simulink model "MSREPrimaryLoop_PlantLevel"  (R2024a)
settings: Solver=VariableStepAuto  StartTime=0.0  StopTime=500000  MaxStep=0.1  RelTol=1e-3
undefined symbols (not defined in the file): a_f, a_g, axialFuelImportance, axialGraphiteImportance, axialPowerFraction, beta, beta_t, bubbleSaturationLevel, bypassRatio, C0, coolantPHXChannelLength, coolantPHXDh, coolantPHXFlowArea, coreCorrectionNominalFlowRate, coreDowncomerArea, coreDowncomerHydraulicDiameter, coreDowncomerLength, coreDowncomerVolume, coreFlowArea, coreFuelVolume, coreInletFlowDistributerArea, coreInletFlowDistributerHydralicDiameter, coreInletFlowDistributerLength, coreInletFlowDistributerVolume, coreLowerPlenumArea, coreLowerPlenumHydraulicDiameter, coreLowerPlenumLength, coreLowerPlenumVolume, coreUpperPlenumArea, coreUpperPlenumLength, coreUpperPlenumVolume, coreVolume, cpGraphite, day, decayScale, decaySSFraction, dissolusionRatio, dMin, dScale, dsmConst, DXeG, externalReactivity, Fiss_factor, fuelChannelHydrualicDiameter, fuelChannelLength, fuelDepositRatio, fuelFraction, fuelGraphiteArea, fuelGraphiteHeatTransferCoefficient, gamma0, gamma1, gamma2, gasExchangeRatio, gasMixingEfficiency, gasPurgeRate, gasStrippingEfficiency, graphiteKDiff, graphiteUnitCellThickness, initialIodineConcentration, InitialXeMolarConcentration ... (+66)
libraries: fl_lib x291, nesl_utility x101, SimscapeFluids_lib x24, simulink x5, slpidlib x1
(part 5 of 13)

== system MSREPrimaryLoop_PlantLevel/Pump MSRE/Pump/PumpPysical ==
  XeIn : Inport
  GasIn : Inport  Port=2
  Add : Sum  Inputs=|++
  Delay One Step : Delay  DelayLength=1
  Gain : Gain  Gain=0.5
  GasCalc : Subsystem
      settings: PortSchema="{\"entries\":[{\"content\":{\"sides\":[{\"content\":{\"connectorIds\":[\"In1\"]},\"type\":\"ConnectorPlacement.EquallySpacedRectSide\",\"uuid\":\"a8e1ce06-71c9-462d-8d5c-7a3e078b5544\"},{\"content\":{\"connectorIds\":[\"Out1\"],\"side\":\"RIGHT\"},\"type\":\"ConnectorPlacement.EquallySpacedRectSide\",\"uuid\":\"2c63a1ce-15e2-4b17-a432-f9f40781bd58\"},{\"content\":{\"connectorIds\":[\"LConn1\",\"LConn2\",\"LConn3\"],\"side\":\"TOP\"},\"type\":\"ConnectorPlacement.EquallySpacedRectSide\",\"uuid\":\"abc20e07-15eb-475f-be7f-cc96378523a1\"},{\"content\":{\"connectorIds\":[],\"side\":\"BOTTOM\"},\"type\":\"ConnectorPlacement.EquallySpacedRectSide\",\"uuid\":\"ab58f362-f4c2-4e86-bda0-802426066295\"}]},\"type\":\"ConnectorPlacement.EquallySpacedConnector\",\"uuid\":\"b54d49a9-048b-4912-bf18-92a7ef5e8aff\"}],\"packageUris\":[\"http://schema.mathworks.com/mf0/Connector/R2020b\"],\"version\":\"1.0\"}"
  PumpPhysics&Control : Subsystem
      settings: PortSchema="{\"entries\":[{\"content\":{\"sides\":[{\"content\":{\"connectorIds\":[\"LConn1\",\"In1\"]},\"type\":\"ConnectorPlacement.EquallySpacedRectSide\",\"uuid\":\"dfa2aa95-b0f6-4d42-b52c-ac64f68b4332\"},{\"content\":{\"connectorIds\":[\"RConn1\"],\"side\":\"RIGHT\"},\"type\":\"ConnectorPlacement.EquallySpacedRectSide\",\"uuid\":\"4e233f45-275b-4a62-b54f-a26261252d76\"},{\"content\":{\"connectorIds\":[],\"side\":\"TOP\"},\"type\":\"ConnectorPlacement.EquallySpacedRectSide\",\"uuid\":\"4d56cee6-54c9-4b53-b595-9dd9843d1812\"},{\"content\":{\"connectorIds\":[\"RConn2\"],\"side\":\"BOTTOM\"},\"type\":\"ConnectorPlacement.EquallySpacedRectSide\",\"uuid\":\"5b59abd0-5c01-4c9b-8b33-a5a665899d43\"}]},\"type\":\"ConnectorPlacement.EquallySpacedConnector\",\"uuid\":\"08118153-6206-4ac8-9187-5e3d4b128de1\"}],\"packageUris\":[\"http://schema.mathworks.com/mf0/Connector/R2020b\"],\"version\":\"1.0\"}"
  XenonCalc : Subsystem
      settings: PortSchema="{\"entries\":[{\"content\":{\"sides\":[{\"content\":{\"connectorIds\":[\"In1\"]},\"type\":\"ConnectorPlacement.EquallySpacedRectSide\",\"uuid\":\"2d0a178d-e3ce-4b60-98e7-1a8cc2d8e60a\"},{\"content\":{\"connectorIds\":[\"Out1\"],\"side\":\"RIGHT\"},\"type\":\"ConnectorPlacement.EquallySpacedRectSide\",\"uuid\":\"c836f1a2-1f60-4759-a54a-d13020949774\"},{\"content\":{\"connectorIds\":[\"LConn1\"],\"side\":\"TOP\"},\"type\":\"ConnectorPlacement.EquallySpacedRectSide\",\"uuid\":\"88d5b9ac-da0a-4ad3-844b-69cd646a8f29\"},{\"content\":{\"connectorIds\":[],\"side\":\"BOTTOM\"},\"type\":\"ConnectorPlacement.EquallySpacedRectSide\",\"uuid\":\"7af8c1ea-1928-402f-ba73-00fd41d484c9\"}]},\"type\":\"ConnectorPlacement.EquallySpacedConnector\",\"uuid\":\"10dc3dbd-7ee0-472f-a356-245132d02761\"}],\"packageUris\":[\"http://schema.mathworks.com/mf0/Connector/R2020b\"],\"version\":\"1.0\"}"
  Inlet : PMIOPort  Side=Left
  Outlet : PMIOPort  Port=2  Side=Right
  XeOut : Outport
  GasOut : Outport  Port=2
  wires:
  GasIn/1 -> GasCalc/1(GasIn), Add/1
  GasCalc/1(GasOut) -> GasOut/1, Add/2
  Add/1 -> Gain/1
  Gain/1 -> Delay One Step/1
  Delay One Step/1 -> PumpPhysics&Control/1(GasRef)
  XeIn/1 -> XenonCalc/1(XeIn)
  XenonCalc/1(XeOut) -> XeOut/1
  connections:
  Inlet/RConn1 -- GasCalc/LConn1 -- PumpPhysics&Control/LConn1
  Outlet/RConn1 -- PumpPhysics&Control/RConn1 -- GasCalc/LConn3
  PumpPhysics&Control/RConn2 -- GasCalc/LConn2 -- XenonCalc/LConn1

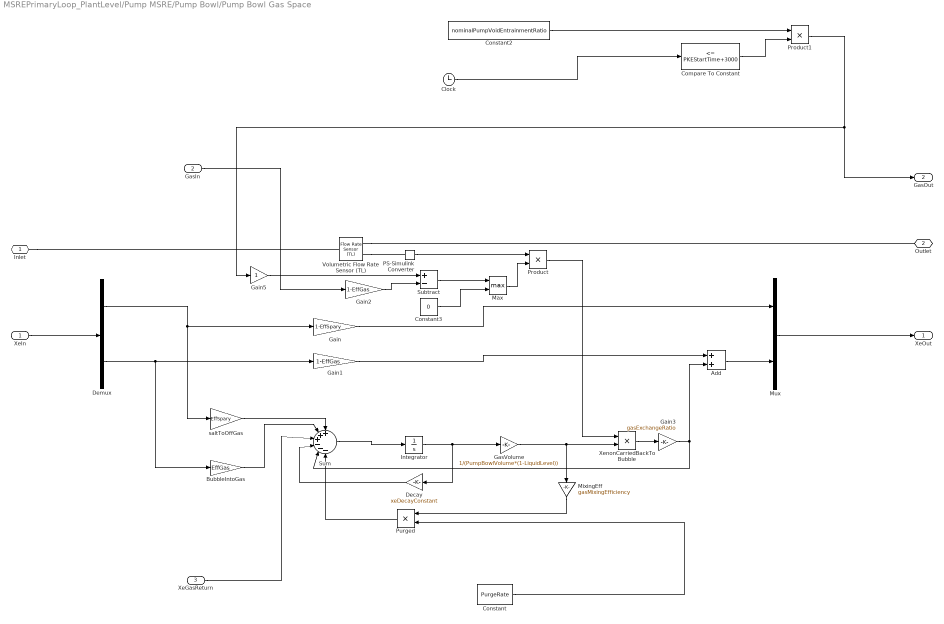
== system MSREPrimaryLoop_PlantLevel/Pump MSRE/Pump Bowl/Pump Bowl Gas Space ==
  XeIn : Inport  OutDataTypeStr=double  Unit=kg/s
  GasIn : Inport  Port=2
  XeGasReturn : Inport  Port=3
  Add : Sum
  BubbleIntoGas : Gain  Gain=EffGas
  Clock : Clock
  Compare To Constant : simulink/Logic and Bit Operations/Compare To Constant  relop=<=  const=PKEStartTime+3000  OutDataTypeStr=boolean
  Constant : Constant  Value=PurgeRate
  Constant2 : Constant  Value=nominalPumpVoidEntrainmentRatio
  Constant3 : Constant  Value=0
  Decay : Gain  Gain=xeDecayConstant
  Demux : Demux  Outputs=2
  Gain : Gain  Gain=1-EffSpary
  Gain1 : Gain  Gain=1-EffGas
  Gain2 : Gain  Gain=1-EffGas
  Gain3 : Gain  Gain=gasExchangeRatio
  Gain5 : Gain
  GasVolume : Gain  Gain=1/(PumpBowlVolume*(1-LiquidLevel))
  Integrator : Integrator  LimitOutput=on  LowerSaturationLimit=0
  Max : MinMax  Function=max  Inputs=2
  MixingEff : Gain  Gain=gasMixingEfficiency
  Mux : Mux  Inputs=2
  PS-Simulink Converter : nesl_utility/PS-Simulink Converter  PhysicalDomain=network_engine_domain  SubClassName=ps_output  LeftPortType=input  RightPortType=output  PseudoPeriodic=off  Frequencies=[]  VectorFormat=1-D array  Unit=inherit  AffineConversion=off
  Product : Product
  Product1 : Product
  Purged : Product
  Subtract : Sum  Inputs=+-
  Sum : Sum  Inputs=+++---
  Volumetric Flow Rate Sensor (TL) : fl_lib/Thermal Liquid/Sensors/Flow Rate Sensor (TL)  mass_flow_measure=false  volumetric_flow_measure=true  energy_flow_measure=false
      settings: InternalSimscapePortConfiguration="{\"Bottom\":[],\"Left\":[{\"id\":\"A\",\"label\":\"A\",\"type\":\"foundation.thermal_liquid.thermal_liquid\"}],\"Right\":[{\"id\":\"B\",\"label\":\"B\",\"type\":\"foundation.thermal_liquid.thermal_liquid\"},{\"id\":\"V\",\"label\":\"V\",\"type\":\"output\"}],\"Top\":[]}"
  XenonCarriedBackToBubble : Product
  saltToOffGas : Gain  Gain=EffSpary
  Inlet : PMIOPort  Side=Left
  Outlet : PMIOPort  Port=2  Side=Right
  XeOut : Outport
  GasOut : Outport  Port=2
  wires:
  XeIn/1 -> Demux/1
  Demux/2 -> Gain1/1, BubbleIntoGas/1
  Mux/1 -> XeOut/1
  Demux/1 -> saltToOffGas/1, Gain/1
  saltToOffGas/1 -> Sum/1
  BubbleIntoGas/1 -> Sum/2
  Integrator/1 -> Decay/1, GasVolume/1
  GasVolume/1 -> XenonCarriedBackToBubble/2, MixingEff/1
  MixingEff/1 -> Purged/1
  Sum/1 -> Integrator/1
  Decay/1 -> Sum/4
  Gain/1 -> Mux/1
  PS-Simulink Converter/1 -> Product/1
  Product/1 -> XenonCarriedBackToBubble/1
  GasIn/1 -> Gain2/1
  Gain1/1 -> Add/1
  Add/1 -> Mux/2
  Product1/1 -> Gain5/1, GasOut/1
  Gain2/1 -> Subtract/2
  Purged/1 -> Sum/6
  XeGasReturn/1 -> Sum/3
  XenonCarriedBackToBubble/1 -> Gain3/1
  Gain3/1 -> Add/2, Sum/5
  Gain5/1 -> Subtract/1
  Subtract/1 -> Max/1
  Max/1 -> Product/2
  Constant3/1 -> Max/2
  Constant/1 -> Purged/2
  Compare To Constant/1 -> Product1/2
  Clock/1 -> Compare To Constant/1
  Constant2/1 -> Product1/1
  connections:
  Inlet/RConn1 -- Volumetric Flow Rate Sensor (TL)/LConn1
  Volumetric Flow Rate Sensor (TL)/RConn1 -- Outlet/RConn1
  Volumetric Flow Rate Sensor (TL)/RConn2 -- PS-Simulink Converter/LConn1

== system MSREPrimaryLoop_PlantLevel/Pump MSRE/Pump Bowl/Salt Space ==
  XeIn : Inport
  GasIn : Inport  Port=2
  Clock : Clock
  Compare To Constant : simulink/Logic and Bit Operations/Compare To Constant  relop=<=  const=PKEStartTime+3000  OutDataTypeStr=boolean
  Constant : Constant  Value=nominalPumpVoidDischargeRatio
  Constant Volume Chamber (TL) : fl_lib/Thermal Liquid/Elements/Constant Volume Chamber (TL)  volume=PumpBowlVolume*LiquidLevel m^3  num_ports=foundation.enum.num_ports.two  area_A=1 m^2  area_B=1 m^2  area_C=0.01 m^2  area_D=0.01 m^2  p_I_specify=on  p_I_priority=High  p_I=P0 Pa  p_I_nominal_specify=off  p_I_nominal_value=1  p_I_nominal_unit=MPa  T_I_specify=on  T_I_priority=None  T_I=T0 K  T_I_nominal_specify=off  T_I_nominal_value=1  T_I_nominal_unit=K  u_I_specify=on  u_I_priority=None  u_I=cpMSRE J/kg  u_I_nominal_specify=off  u_I_nominal_value=1  u_I_nominal_unit=kJ/kg  rho_I_specify=on  rho_I_priority=None  rho_I=nominalFuelDensity kg/m^3  rho_I_nominal_specify=off  rho_I_nominal_value=1  rho_I_nominal_unit=kg/m^3
      settings: InternalSimscapePortConfiguration="{\"Bottom\":[],\"Left\":[{\"id\":\"A\",\"label\":\"A\",\"type\":\"foundation.thermal_liquid.thermal_liquid\"},{\"id\":\"H\",\"label\":\"H\",\"type\":\"foundation.thermal.thermal\"}],\"Right\":[{\"id\":\"B\",\"label\":\"B\",\"type\":\"foundation.thermal_liquid.thermal_liquid\"}],\"Top\":[]}"
  GasCalc : Subsystem  mask{PipeVolume=PumpBowlVolume*LiquidLevel}
      mask prompts: PipeVolume "Volume"
      settings: PortSchema="{\"entries\":[{\"content\":{\"sides\":[{\"content\":{\"connectorIds\":[\"In1\"]},\"type\":\"ConnectorPlacement.EquallySpacedRectSide\",\"uuid\":\"a8e1ce06-71c9-462d-8d5c-7a3e078b5544\"},{\"content\":{\"connectorIds\":[\"Out1\"],\"side\":\"RIGHT\"},\"type\":\"ConnectorPlacement.EquallySpacedRectSide\",\"uuid\":\"2c63a1ce-15e2-4b17-a432-f9f40781bd58\"},{\"content\":{\"connectorIds\":[\"LConn1\"],\"side\":\"TOP\"},\"type\":\"ConnectorPlacement.EquallySpacedRectSide\",\"uuid\":\"abc20e07-15eb-475f-be7f-cc96378523a1\"},{\"content\":{\"connectorIds\":[],\"side\":\"BOTTOM\"},\"type\":\"ConnectorPlacement.EquallySpacedRectSide\",\"uuid\":\"ab58f362-f4c2-4e86-bda0-802426066295\"}]},\"type\":\"ConnectorPlacement.EquallySpacedConnector\",\"uuid\":\"b54d49a9-048b-4912-bf18-92a7ef5e8aff\"}],\"packageUris\":[\"http://schema.mathworks.com/mf0/Connector/R2020b\"],\"version\":\"1.0\"}"
  Perfect Insulator : fl_lib/Thermal/Thermal Elements/Perfect Insulator  T_specify=off  T_priority=None  T=0 K  T_nominal_specify=off  T_nominal_value=1  T_nominal_unit=K
  Product1 : Product
  Volumetric Flow Rate Sensor (TL) : fl_lib/Thermal Liquid/Sensors/Flow Rate Sensor (TL)  mass_flow_measure=false  volumetric_flow_measure=true  energy_flow_measure=false
      settings: InternalSimscapePortConfiguration="{\"Bottom\":[],\"Left\":[{\"id\":\"A\",\"label\":\"A\",\"type\":\"foundation.thermal_liquid.thermal_liquid\"}],\"Right\":[{\"id\":\"B\",\"label\":\"B\",\"type\":\"foundation.thermal_liquid.thermal_liquid\"},{\"id\":\"V\",\"label\":\"V\",\"type\":\"output\"}],\"Top\":[]}"
  XenonCalcBowl : Subsystem  mask{PipeVolume=PumpBowlVolume*LiquidLevel, dsm=0.005*dScale, km=0.0001}
      mask prompts: PipeVolume "Volume"; dsm "Sauter Mean Diameter"; km "Mass Transfer Coefficient"
      settings: PortSchema="{\"entries\":[{\"content\":{\"sides\":[{\"content\":{\"connectorIds\":[\"LConn1\",\"In1\",\"In2\"]},\"type\":\"ConnectorPlacement.EquallySpacedRectSide\",\"uuid\":\"82f8e7e7-fd89-4597-952e-64db268d0190\"},{\"content\":{\"connectorIds\":[\"RConn1\",\"Out1\",\"Out2\"],\"side\":\"RIGHT\"},\"type\":\"ConnectorPlacement.EquallySpacedRectSide\",\"uuid\":\"4b3edad1-18f8-43fa-96ee-a24bb3384b59\"},{\"content\":{\"connectorIds\":[],\"side\":\"TOP\"},\"type\":\"ConnectorPlacement.EquallySpacedRectSide\",\"uuid\":\"43d4f51d-f841-40d6-804e-7f238a90dabe\"},{\"content\":{\"connectorIds\":[],\"side\":\"BOTTOM\"},\"type\":\"ConnectorPlacement.EquallySpacedRectSide\",\"uuid\":\"350f2274-4108-4e6e-a637-0ae7118de3f0\"}]},\"type\":\"ConnectorPlacement.EquallySpacedConnector\",\"uuid\":\"d7e795ea-9d5d-4a8c-83ab-dab42197cc2f\"}],\"packageUris\":[\"http://schema.mathworks.com/mf0/Connector/R2020b\"],\"version\":\"1.0\"}"
  Inlet : PMIOPort  Side=Left
  Outlet : PMIOPort  Port=2  Side=Right
  XeOut : Outport
  GasOut : Outport  Port=2
  XeGasReturn : Outport  Port=3
  wires:
  XeIn/1 -> XenonCalcBowl/1(XeIn)
  XenonCalcBowl/1(XeOut) -> XeOut/1
  GasIn/1 -> GasCalc/1(GasIn)
  GasCalc/1(AverageVoid) -> XenonCalcBowl/2(GasVoid)
  XenonCalcBowl/2(XeGasReturn) -> XeGasReturn/1
  Product1/1 -> GasOut/1
  Compare To Constant/1 -> Product1/2
  Clock/1 -> Compare To Constant/1
  Constant/1 -> Product1/1
  connections:
  XenonCalcBowl/LConn1 -- Volumetric Flow Rate Sensor (TL)/RConn1
  Volumetric Flow Rate Sensor (TL)/LConn1 -- Inlet/RConn1
  XenonCalcBowl/RConn1 -- Constant Volume Chamber (TL)/LConn1
  Constant Volume Chamber (TL)/RConn1 -- Outlet/RConn1
  Perfect Insulator/LConn1 -- Constant Volume Chamber (TL)/LConn2
  GasCalc/LConn1 -- Volumetric Flow Rate Sensor (TL)/RConn2

== system MSREPrimaryLoop_PlantLevel/Pump MSRE/Pump Flow Distribution/Subsystem1 ==
  note: Handle divide by zero.
  MainXeRate : fl_lib/Physical Signals/Functions/PS Divide
  Mass & Energy Flow Rate Sensor (TL) : fl_lib/Thermal Liquid/Sensors/Flow Rate Sensor (TL)  mass_flow_measure=true  volumetric_flow_measure=false  energy_flow_measure=true
      settings: InternalSimscapePortConfiguration="{\"Bottom\":[{\"id\":\"PHI\",\"label\":\"φ\",\"type\":\"output\"}],\"Left\":[{\"id\":\"A\",\"label\":\"A\",\"type\":\"foundation.thermal_liquid.thermal_liquid\"}],\"Right\":[{\"id\":\"B\",\"label\":\"B\",\"type\":\"foundation.thermal_liquid.thermal_liquid\"},{\"id\":\"M\",\"label\":\"M\",\"type\":\"output\"}],\"Top\":[]}"
  Mass & Energy Flow Rate Sensor (TL)1 : fl_lib/Thermal Liquid/Sensors/Flow Rate Sensor (TL)  mass_flow_measure=true  volumetric_flow_measure=false  energy_flow_measure=true
      settings: InternalSimscapePortConfiguration="{\"Bottom\":[{\"id\":\"PHI\",\"label\":\"φ\",\"type\":\"output\"}],\"Left\":[{\"id\":\"A\",\"label\":\"A\",\"type\":\"foundation.thermal_liquid.thermal_liquid\"}],\"Right\":[{\"id\":\"B\",\"label\":\"B\",\"type\":\"foundation.thermal_liquid.thermal_liquid\"},{\"id\":\"M\",\"label\":\"M\",\"type\":\"output\"}],\"Top\":[]}"
  Mass & Energy Flow Rate Sensor (TL)2 : fl_lib/Thermal Liquid/Sensors/Flow Rate Sensor (TL)  mass_flow_measure=true  volumetric_flow_measure=false  energy_flow_measure=true
      settings: InternalSimscapePortConfiguration="{\"Bottom\":[{\"id\":\"PHI\",\"label\":\"φ\",\"type\":\"output\"}],\"Left\":[{\"id\":\"A\",\"label\":\"A\",\"type\":\"foundation.thermal_liquid.thermal_liquid\"}],\"Right\":[{\"id\":\"B\",\"label\":\"B\",\"type\":\"foundation.thermal_liquid.thermal_liquid\"},{\"id\":\"M\",\"label\":\"M\",\"type\":\"output\"}],\"Top\":[]}"
  PS Abs : fl_lib/Physical Signals/Nonlinear Operators/PS Abs
      settings: InternalSimscapePortConfiguration="{\"Bottom\":[],\"Left\":[{\"id\":\"I\",\"label\":\"\",\"type\":\"input\"}],\"Right\":[{\"id\":\"O\",\"label\":\"\",\"type\":\"output\"}],\"Top\":[]}"
  PS Abs1 : fl_lib/Physical Signals/Nonlinear Operators/PS Abs
      settings: InternalSimscapePortConfiguration="{\"Bottom\":[],\"Left\":[{\"id\":\"I\",\"label\":\"\",\"type\":\"input\"}],\"Right\":[{\"id\":\"O\",\"label\":\"\",\"type\":\"output\"}],\"Top\":[]}"
  PS Abs2 : fl_lib/Physical Signals/Nonlinear Operators/PS Abs
      settings: InternalSimscapePortConfiguration="{\"Bottom\":[],\"Left\":[{\"id\":\"I\",\"label\":\"\",\"type\":\"input\"}],\"Right\":[{\"id\":\"O\",\"label\":\"\",\"type\":\"output\"}],\"Top\":[]}"
  PS Constant : fl_lib/Physical Signals/Sources/PS Constant  constant=1e-6 kg/s
  PS Max : fl_lib/Physical Signals/Nonlinear Operators/PS Max
      settings: InternalSimscapePortConfiguration="{\"Bottom\":[],\"Left\":[{\"id\":\"I1\",\"label\":\"\",\"type\":\"input\"},{\"id\":\"I2\",\"label\":\"\",\"type\":\"input\"}],\"Right\":[{\"id\":\"O\",\"label\":\"\",\"type\":\"output\"}],\"Top\":[]}"
  PS-Simulink Converter : nesl_utility/PS-Simulink Converter  PhysicalDomain=network_engine_domain  SubClassName=ps_output  LeftPortType=input  RightPortType=output  PseudoPeriodic=off  Frequencies=[]  VectorFormat=1-D array  Unit=inherit  AffineConversion=off
  PS-Simulink Converter2 : nesl_utility/PS-Simulink Converter  PhysicalDomain=network_engine_domain  SubClassName=ps_output  LeftPortType=input  RightPortType=output  PseudoPeriodic=off  Frequencies=[]  VectorFormat=1-D array  Unit=inherit  AffineConversion=off
  SideXeRate : fl_lib/Physical Signals/Functions/PS Divide
  Subsystem : Subsystem  mask{byPassRatio=sprayFlowRate/(VDot+sprayFlowRate)}
      mask prompts: byPassRatio "By Pass Ratio"
  Inlet : PMIOPort  Side=Left
  MainOut : PMIOPort  Port=2  Side=Right
  SideOut : PMIOPort  Port=3  Side=Right
  MainRatio : Outport
  SideRatio : Outport  Port=2
  wires:
  PS-Simulink Converter2/1 -> MainRatio/1
  PS-Simulink Converter/1 -> SideRatio/1
  connections:
  MainXeRate/LConn1 -- PS Abs2/RConn1
  Mass & Energy Flow Rate Sensor (TL)/RConn1 -- Subsystem/LConn1
  Mass & Energy Flow Rate Sensor (TL)1/RConn1 -- SideOut/RConn1
  Mass & Energy Flow Rate Sensor (TL)1/RConn2 -- PS Abs1/LConn1
  Mass & Energy Flow Rate Sensor (TL)1/LConn1 -- Subsystem/RConn2
  PS Abs/RConn1 -- PS Max/LConn1
  PS Constant/RConn1 -- PS Max/LConn2
  PS Abs1/RConn1 -- SideXeRate/LConn1
  MainXeRate/RConn1 -- PS-Simulink Converter2/LConn1
  PS Abs2/LConn1 -- Mass & Energy Flow Rate Sensor (TL)2/RConn2
  SideXeRate/RConn1 -- PS-Simulink Converter/LConn1
  PS Max/RConn1 -- MainXeRate/LConn2 -- SideXeRate/LConn2
  Mass & Energy Flow Rate Sensor (TL)/RConn2 -- PS Abs/LConn1
  Mass & Energy Flow Rate Sensor (TL)2/LConn1 -- Subsystem/RConn1
  Mass & Energy Flow Rate Sensor (TL)/LConn1 -- Inlet/RConn1
  Mass & Energy Flow Rate Sensor (TL)2/RConn1 -- MainOut/RConn1

== system MSREPrimaryLoop_PlantLevel/Reactor/CoreTH&Inerti/Core ==
  XeIn : Inport
  GasIn : Inport  Port=2
  IodineSNumberDensity : Inport  Port=3
  NeutronFraction : Inport  Port=4
  DecayFraction : Inport  Port=5
  CoreTH : Subsystem  mask{N_nodes=4, FuelDepositRatio=fuelDepositRatio, k_graphite=kGraphite, cp_graphite=cpGraphite, rho_graphite=rhoGraphite, UnitCellGraphiteThickness=graphiteUnitCellThickness, h_fg=fuelGraphiteHeatTransferCoefficient, T0=T0, P0=P0}
      mask prompts: N_nodes "Number Of Nodes"; k_graphite "Graphite Thermal Conductivity"; cp_graphite "Graphite Specific Thermal Capacity"; rho_graphite "Graphite Density"; UnitCellGraphiteThickness "Unit Cell Graphite Thickness"; h_fg "Fuel Graphite Heat Transfer Coefficient"; T0 "Initial Temperature"; P0 "Initial Pressure"
      settings: PortSchema="{\"entries\":[{\"content\":{\"sides\":[{\"content\":{\"connectorIds\":[\"LConn1\",\"LConn2\",\"LConn3\"]},\"type\":\"ConnectorPlacement.EquallySpacedRectSide\",\"uuid\":\"1c20b62e-1aca-4cc3-9434-4d9ffc0779e4\"},{\"content\":{\"connectorIds\":[\"Out1\",\"RConn1\"],\"side\":\"RIGHT\"},\"type\":\"ConnectorPlacement.EquallySpacedRectSide\",\"uuid\":\"cbe92cdf-09f7-4580-a6a7-168080192112\"},{\"content\":{\"connectorIds\":[\"In1\",\"In2\"],\"side\":\"TOP\"},\"type\":\"ConnectorPlacement.EquallySpacedRectSide\",\"uuid\":\"70a4d7aa-1432-4349-89f0-42a0194e580f\"},{\"content\":{\"connectorIds\":[\"In3\"],\"side\":\"BOTTOM\"},\"type\":\"ConnectorPlacement.EquallySpacedRectSide\",\"uuid\":\"7c92aed1-92dd-461a-937a-8dd840527e94\"}]},\"type\":\"ConnectorPlacement.EquallySpacedConnector\",\"uuid\":\"1a67b279-14f5-41a4-8cd2-abe76a0f00c3\"}],\"packageUris\":[\"http://schema.mathworks.com/mf0/Connector/R2020b\"],\"version\":\"1.0\"}"
  CoreXenonCalc : Subsystem
      settings: PortSchema="{\"entries\":[{\"content\":{\"sides\":[{\"content\":{\"connectorIds\":[\"In1\",\"LConn1\"]},\"type\":\"ConnectorPlacement.EquallySpacedRectSide\",\"uuid\":\"82f8e7e7-fd89-4597-952e-64db268d0190\"},{\"content\":{\"connectorIds\":[\"Out1\",\"Out2\",\"RConn1\"],\"side\":\"RIGHT\"},\"type\":\"ConnectorPlacement.EquallySpacedRectSide\",\"uuid\":\"4b3edad1-18f8-43fa-96ee-a24bb3384b59\"},{\"content\":{\"connectorIds\":[\"In2\",\"In3\",\"In4\"],\"side\":\"TOP\"},\"type\":\"ConnectorPlacement.EquallySpacedRectSide\",\"uuid\":\"43d4f51d-f841-40d6-804e-7f238a90dabe\"},{\"content\":{\"connectorIds\":[\"In5\",\"In6\"],\"side\":\"BOTTOM\"},\"type\":\"ConnectorPlacement.EquallySpacedRectSide\",\"uuid\":\"350f2274-4108-4e6e-a637-0ae7118de3f0\"}]},\"type\":\"ConnectorPlacement.EquallySpacedConnector\",\"uuid\":\"d7e795ea-9d5d-4a8c-83ab-dab42197cc2f\"}],\"packageUris\":[\"http://schema.mathworks.com/mf0/Connector/R2020b\"],\"version\":\"1.0\"}"
  Delay One Step : Delay  DelayLength=1  InitialCondition=T0
  PLossFunc : Subsystem
      settings: PortSchema="{\"entries\":[{\"content\":{\"sides\":[{\"content\":{\"connectorIds\":[\"Out1\",\"LConn1\"]},\"type\":\"ConnectorPlacement.EquallySpacedRectSide\",\"uuid\":\"95ca4545-c473-4e31-844b-c43557042c16\"},{\"content\":{\"connectorIds\":[\"RConn1\"],\"side\":\"RIGHT\"},\"type\":\"ConnectorPlacement.EquallySpacedRectSide\",\"uuid\":\"f9304c30-8684-4a05-a34b-3121610e628d\"},{\"content\":{\"connectorIds\":[],\"side\":\"TOP\"},\"type\":\"ConnectorPlacement.EquallySpacedRectSide\",\"uuid\":\"64c7a4d8-8539-4303-ae81-4015bd1451af\"}]},\"type\":\"ConnectorPlacement.EquallySpacedConnector\",\"uuid\":\"40c12b2f-fb9d-4a19-b6f1-e93ae1fd4d68\"}],\"packageUris\":[\"http://schema.mathworks.com/mf0/Connector/R2020b\"],\"version\":\"1.0\"}"
  SolubilityReduction : Subsystem
      settings: PortSchema="{\"entries\":[{\"content\":{\"sides\":[{\"content\":{\"connectorIds\":[\"In1\",\"In2\"]},\"type\":\"ConnectorPlacement.EquallySpacedRectSide\",\"uuid\":\"faacc406-4069-496b-af99-41d2aed9dfc2\"},{\"content\":{\"connectorIds\":[\"Out1\",\"Out2\",\"Out3\"],\"side\":\"RIGHT\"},\"type\":\"ConnectorPlacement.EquallySpacedRectSide\",\"uuid\":\"94f1539c-5515-4bd6-bffb-3a5caf43f7b6\"},{\"content\":{\"connectorIds\":[],\"side\":\"TOP\"},\"type\":\"ConnectorPlacement.EquallySpacedRectSide\",\"uuid\":\"d17dce47-2058-4206-8706-4dc771d04045\"},{\"content\":{\"connectorIds\":[\"Out4\"],\"side\":\"BOTTOM\"},\"type\":\"ConnectorPlacement.EquallySpacedRectSide\",\"uuid\":\"97529780-84fa-4776-a404-e5a3e7258a40\"}]},\"type\":\"ConnectorPlacement.EquallySpacedConnector\",\"uuid\":\"1ce9374c-8c3e-43ec-9da7-5b483b5e3d48\"}],\"packageUris\":[\"http://schema.mathworks.com/mf0/Connector/R2020b\"],\"version\":\"1.0\"}"
  Subsystem : Subsystem
  Subsystem1 : Subsystem
      settings: PortSchema="{\"entries\":[{\"content\":{\"sides\":[{\"content\":{\"connectorIds\":[\"In1\",\"In2\"]},\"type\":\"ConnectorPlacement.EquallySpacedRectSide\",\"uuid\":\"2a068eb5-92e4-43e3-b748-0f561ebb2f0e\"},{\"content\":{\"connectorIds\":[\"Out1\",\"Out2\"],\"side\":\"RIGHT\"},\"type\":\"ConnectorPlacement.EquallySpacedRectSide\",\"uuid\":\"d07e14f8-d0ba-4d92-9a78-613216e777c8\"},{\"content\":{\"connectorIds\":[\"LConn1\",\"LConn2\",\"Out3\",\"LConn3\"],\"side\":\"TOP\"},\"type\":\"ConnectorPlacement.EquallySpacedRectSide\",\"uuid\":\"40c9f9fd-9b75-4721-9a62-c538b0ea8b4c\"}]},\"type\":\"ConnectorPlacement.EquallySpacedConnector\",\"uuid\":\"1283fec4-e55b-4051-bba7-bc8dde4dc12d\"}],\"packageUris\":[\"http://schema.mathworks.com/mf0/Connector/R2020b\"],\"version\":\"1.0\"}"
  Subsystem2 : Subsystem  Variant=on  VariantControlMode=label  VariantControl=Choice  LabelModeActiveChoice=Constant
      settings: PortSchema="{\"entries\":[{\"content\":{\"sides\":[{\"content\":{\"connectorIds\":[\"In1\",\"In2\",\"In3\"]},\"type\":\"ConnectorPlacement.EquallySpacedRectSide\",\"uuid\":\"cfe1ce7c-1611-431e-9412-2b3caba343b3\"},{\"content\":{\"connectorIds\":[\"Out1\",\"Out2\"],\"side\":\"RIGHT\"},\"type\":\"ConnectorPlacement.EquallySpacedRectSide\",\"uuid\":\"0c689a27-e89a-4b17-8ea0-ad5769387ae3\"},{\"content\":{\"connectorIds\":[\"In4\"],\"side\":\"TOP\"},\"type\":\"ConnectorPlacement.EquallySpacedRectSide\",\"uuid\":\"a650924a-5c90-44bf-97de-77f017d49b56\"},{\"content\":{\"connectorIds\":[\"In5\"],\"side\":\"BOTTOM\"},\"type\":\"ConnectorPlacement.EquallySpacedRectSide\",\"uuid\":\"af91b143-b368-4d0c-8cc7-2ed084fb2df7\"}]},\"type\":\"ConnectorPlacement.EquallySpacedConnector\",\"uuid\":\"a7e506ef-3f33-4307-859c-c22ba4b969e5\"}],\"packageUris\":[\"http://schema.mathworks.com/mf0/Connector/R2020b\"],\"version\":\"1.0\"}"
  Volumetric Flow Rate Sensor (TL) : fl_lib/Thermal Liquid/Sensors/Flow Rate Sensor (TL)  mass_flow_measure=false  volumetric_flow_measure=true  energy_flow_measure=false
      settings: InternalSimscapePortConfiguration="{\"Bottom\":[],\"Left\":[{\"id\":\"A\",\"label\":\"A\",\"type\":\"foundation.thermal_liquid.thermal_liquid\"}],\"Right\":[{\"id\":\"B\",\"label\":\"B\",\"type\":\"foundation.thermal_liquid.thermal_liquid\"},{\"id\":\"V\",\"label\":\"V\",\"type\":\"output\"}],\"Top\":[]}"
  Inlet : PMIOPort  Side=Left
  InletSideHeatTranfser : PMIOPort  Port=2  Side=Left
  Outlet : PMIOPort  Port=3  Side=Right
  " Outlet Side Heat Transfer" : PMIOPort  Port=4  Side=Right
  XeOut : Outport
  GasOut : Outport  Port=2
  "TotalXeCrossSection, [cm^2]" : Outport  Port=3
  Temperatures : Outport  Port=4
  wires:
  NeutronFraction/1 -> CoreTH/2(NeutronFraction), CoreXenonCalc/4(NeutronFraction)
  CoreTH/1(Temperatures) -> Temperatures/1, Subsystem/1(Temperatures)
  XeIn/1 -> SolubilityReduction/1(XeIn)
  Delay One Step/1 -> CoreXenonCalc/3(T_f_ave), Subsystem2/4(Temperature)
  CoreXenonCalc/2("TotalXeCrossSection, [cm^2]") -> "TotalXeCrossSection, [cm^2]"/1
  Subsystem/1(T_f_ave) -> Delay One Step/1
  IodineSNumberDensity/1 -> CoreXenonCalc/2(IodineSNumberDensity)
  SolubilityReduction/1(XeOut) -> CoreXenonCalc/1(XeIn)
  GasIn/1 -> SolubilityReduction/2(GasIn)
  DecayFraction/1 -> CoreTH/1(DecayFraction)
  Subsystem1/3(GasRefOut) -> CoreTH/3(GasRef), CoreXenonCalc/6(GasRef)
  SolubilityReduction/2(GasOut) -> Subsystem1/1(GasIn)
  SolubilityReduction/3(AbsorbedGas) -> Subsystem1/2(Absorbed)
  PLossFunc/1(PLoss) -> CoreXenonCalc/5(PLoss)
  CoreXenonCalc/1(XeOut) -> Subsystem2/1(XeIn)
  Subsystem1/1(GasOut) -> Subsystem2/2(GasIn)
  Subsystem1/2(AbsorbedOut) -> Subsystem2/3(AbsorbedOut)
  SolubilityReduction/4(ModeSwitch) -> Subsystem2/5(ModeSwitch)
  Subsystem2/1(GasOut) -> GasOut/1
  Subsystem2/2(XeOut) -> XeOut/1
  connections:
  Volumetric Flow Rate Sensor (TL)/LConn1 -- PLossFunc/LConn1 -- Subsystem1/LConn1 -- Inlet/RConn1
  Volumetric Flow Rate Sensor (TL)/RConn1 -- CoreXenonCalc/LConn1
  CoreXenonCalc/RConn1 -- CoreTH/LConn1
  CoreTH/RConn1 -- Outlet/RConn1 -- PLossFunc/RConn1 -- Subsystem1/LConn3
  Volumetric Flow Rate Sensor (TL)/RConn2 -- Subsystem1/LConn2
  CoreTH/LConn2 -- InletSideHeatTranfser/RConn1
  CoreTH/LConn3 -- " Outlet Side Heat Transfer"/RConn1

== system MSREPrimaryLoop_PlantLevel/Reactor/CoreTH&Inerti/DownComer ==
  XeIn : Inport
  GasIn : Inport  Port=2
  Add : Sum  Inputs=|++
  Delay One Step : Delay  DelayLength=1
  Downcomer : Subsystem
      settings: PortSchema="{\"entries\":[{\"content\":{\"sides\":[{\"content\":{\"connectorIds\":[\"LConn1\",\"In1\"]},\"type\":\"ConnectorPlacement.EquallySpacedRectSide\",\"uuid\":\"0f255306-ec83-4423-ac41-a2708bd1ec44\"},{\"content\":{\"connectorIds\":[\"RConn1\",\"RConn2\"],\"side\":\"RIGHT\"},\"type\":\"ConnectorPlacement.EquallySpacedRectSide\",\"uuid\":\"650fb4ea-7b32-4c45-8538-9785d9ca64bf\"},{\"content\":{\"connectorIds\":[],\"side\":\"TOP\"},\"type\":\"ConnectorPlacement.EquallySpacedRectSide\",\"uuid\":\"434d3568-54a4-4787-a287-69f15ef478cb\"},{\"content\":{\"connectorIds\":[\"RConn3\"],\"side\":\"BOTTOM\"},\"type\":\"ConnectorPlacement.EquallySpacedRectSide\",\"uuid\":\"5b0b510d-1175-4508-bbe9-65b563e28484\"}]},\"type\":\"ConnectorPlacement.EquallySpacedConnector\",\"uuid\":\"b18d9c84-3d71-444b-a89d-79c3dc70d4d9\"}],\"packageUris\":[\"http://schema.mathworks.com/mf0/Connector/R2020b\"],\"version\":\"1.0\"}"
  Gain : Gain  Gain=0.5
  GasCalc : Subsystem  mask{Volume=Volume}
      settings: PortSchema="{\"entries\":[{\"content\":{\"sides\":[{\"content\":{\"connectorIds\":[\"In1\"]},\"type\":\"ConnectorPlacement.EquallySpacedRectSide\",\"uuid\":\"a8e1ce06-71c9-462d-8d5c-7a3e078b5544\"},{\"content\":{\"connectorIds\":[\"Out1\"],\"side\":\"RIGHT\"},\"type\":\"ConnectorPlacement.EquallySpacedRectSide\",\"uuid\":\"2c63a1ce-15e2-4b17-a432-f9f40781bd58\"},{\"content\":{\"connectorIds\":[\"LConn1\",\"LConn2\",\"LConn3\"],\"side\":\"TOP\"},\"type\":\"ConnectorPlacement.EquallySpacedRectSide\",\"uuid\":\"abc20e07-15eb-475f-be7f-cc96378523a1\"},{\"content\":{\"connectorIds\":[],\"side\":\"BOTTOM\"},\"type\":\"ConnectorPlacement.EquallySpacedRectSide\",\"uuid\":\"ab58f362-f4c2-4e86-bda0-802426066295\"}]},\"type\":\"ConnectorPlacement.EquallySpacedConnector\",\"uuid\":\"b54d49a9-048b-4912-bf18-92a7ef5e8aff\"}],\"packageUris\":[\"http://schema.mathworks.com/mf0/Connector/R2020b\"],\"version\":\"1.0\"}"
  PLossFunc : Subsystem
      settings: PortSchema="{\"entries\":[{\"content\":{\"sides\":[{\"content\":{\"connectorIds\":[\"Out1\",\"LConn1\"]},\"type\":\"ConnectorPlacement.EquallySpacedRectSide\",\"uuid\":\"95ca4545-c473-4e31-844b-c43557042c16\"},{\"content\":{\"connectorIds\":[\"RConn1\"],\"side\":\"RIGHT\"},\"type\":\"ConnectorPlacement.EquallySpacedRectSide\",\"uuid\":\"f9304c30-8684-4a05-a34b-3121610e628d\"},{\"content\":{\"connectorIds\":[],\"side\":\"TOP\"},\"type\":\"ConnectorPlacement.EquallySpacedRectSide\",\"uuid\":\"64c7a4d8-8539-4303-ae81-4015bd1451af\"}]},\"type\":\"ConnectorPlacement.EquallySpacedConnector\",\"uuid\":\"40c12b2f-fb9d-4a19-b6f1-e93ae1fd4d68\"}],\"packageUris\":[\"http://schema.mathworks.com/mf0/Connector/R2020b\"],\"version\":\"1.0\"}"
  XenonCalc : Subsystem  mask{Volume=Volume, Area=Area, Length=Length, Dh=Dh, Elevation=Elevation}
      mask prompts: Dh "Hydraulic Diameter"
      settings: PortSchema="{\"entries\":[{\"content\":{\"sides\":[{\"content\":{\"connectorIds\":[\"LConn1\",\"In1\"]},\"type\":\"ConnectorPlacement.EquallySpacedRectSide\",\"uuid\":\"82f8e7e7-fd89-4597-952e-64db268d0190\"},{\"content\":{\"connectorIds\":[\"RConn1\",\"Out1\"],\"side\":\"RIGHT\"},\"type\":\"ConnectorPlacement.EquallySpacedRectSide\",\"uuid\":\"4b3edad1-18f8-43fa-96ee-a24bb3384b59\"},{\"content\":{\"connectorIds\":[\"In2\"],\"side\":\"TOP\"},\"type\":\"ConnectorPlacement.EquallySpacedRectSide\",\"uuid\":\"43d4f51d-f841-40d6-804e-7f238a90dabe\"},{\"content\":{\"connectorIds\":[\"In3\"],\"side\":\"BOTTOM\"},\"type\":\"ConnectorPlacement.EquallySpacedRectSide\",\"uuid\":\"350f2274-4108-4e6e-a637-0ae7118de3f0\"}]},\"type\":\"ConnectorPlacement.EquallySpacedConnector\",\"uuid\":\"d7e795ea-9d5d-4a8c-83ab-dab42197cc2f\"}],\"packageUris\":[\"http://schema.mathworks.com/mf0/Connector/R2020b\"],\"version\":\"1.0\"}"
  Inlet : PMIOPort  Side=Left
  Outlet : PMIOPort  Port=2  Side=Right
  Thermal : PMIOPort  Port=3  Side=Left
  XeOut : Outport
  GasOut : Outport  Port=2
  wires:
  XenonCalc/1(XeOut) -> XeOut/1
  Add/1 -> Gain/1
  GasCalc/1(GasOut) -> GasOut/1, Add/2
  Gain/1 -> Delay One Step/1
  GasIn/1 -> GasCalc/1(GasIn), Add/1
  Delay One Step/1 -> XenonCalc/3(GasRef), Downcomer/1(GasInRef)
  XeIn/1 -> XenonCalc/1(XeIn)
  PLossFunc/1(PLoss) -> XenonCalc/2(PLoss)
  connections:
  Inlet/RConn1 -- GasCalc/LConn1 -- XenonCalc/LConn1
  Outlet/RConn1 -- PLossFunc/RConn1 -- GasCalc/LConn3 -- Downcomer/RConn2
  GasCalc/LConn2 -- Downcomer/RConn3
  XenonCalc/RConn1 -- PLossFunc/LConn1 -- Downcomer/LConn1
  Downcomer/RConn1 -- Thermal/RConn1

== system MSREPrimaryLoop_PlantLevel/Reactor/CoreTH&Inerti/Inlet Distribution ==
  XeIn : Inport
  GasIn : Inport  Port=2
  Add : Sum  Inputs=|++
  Delay One Step : Delay  DelayLength=1
  Gain : Gain  Gain=0.5
  GasCalc : Subsystem  mask{Volume=Volume}
      settings: PortSchema="{\"entries\":[{\"content\":{\"sides\":[{\"content\":{\"connectorIds\":[\"In1\"]},\"type\":\"ConnectorPlacement.EquallySpacedRectSide\",\"uuid\":\"a8e1ce06-71c9-462d-8d5c-7a3e078b5544\"},{\"content\":{\"connectorIds\":[\"Out1\"],\"side\":\"RIGHT\"},\"type\":\"ConnectorPlacement.EquallySpacedRectSide\",\"uuid\":\"2c63a1ce-15e2-4b17-a432-f9f40781bd58\"},{\"content\":{\"connectorIds\":[\"LConn1\",\"LConn2\",\"LConn3\"],\"side\":\"TOP\"},\"type\":\"ConnectorPlacement.EquallySpacedRectSide\",\"uuid\":\"abc20e07-15eb-475f-be7f-cc96378523a1\"},{\"content\":{\"connectorIds\":[],\"side\":\"BOTTOM\"},\"type\":\"ConnectorPlacement.EquallySpacedRectSide\",\"uuid\":\"ab58f362-f4c2-4e86-bda0-802426066295\"}]},\"type\":\"ConnectorPlacement.EquallySpacedConnector\",\"uuid\":\"b54d49a9-048b-4912-bf18-92a7ef5e8aff\"}],\"packageUris\":[\"http://schema.mathworks.com/mf0/Connector/R2020b\"],\"version\":\"1.0\"}"
  InletDistributor : Subsystem
      settings: PortSchema="{\"entries\":[{\"content\":{\"sides\":[{\"content\":{\"connectorIds\":[\"LConn1\",\"In1\"]},\"type\":\"ConnectorPlacement.EquallySpacedRectSide\",\"uuid\":\"0f255306-ec83-4423-ac41-a2708bd1ec44\"},{\"content\":{\"connectorIds\":[\"RConn1\"],\"side\":\"RIGHT\"},\"type\":\"ConnectorPlacement.EquallySpacedRectSide\",\"uuid\":\"650fb4ea-7b32-4c45-8538-9785d9ca64bf\"},{\"content\":{\"side\":\"TOP\"},\"type\":\"ConnectorPlacement.EquallySpacedRectSide\",\"uuid\":\"434d3568-54a4-4787-a287-69f15ef478cb\"},{\"content\":{\"connectorIds\":[\"RConn2\"],\"side\":\"BOTTOM\"},\"type\":\"ConnectorPlacement.EquallySpacedRectSide\",\"uuid\":\"5b0b510d-1175-4508-bbe9-65b563e28484\"}]},\"type\":\"ConnectorPlacement.EquallySpacedConnector\",\"uuid\":\"b18d9c84-3d71-444b-a89d-79c3dc70d4d9\"}],\"packageUris\":[\"http://schema.mathworks.com/mf0/Connector/R2020b\"],\"version\":\"1.0\"}"
  PLossFunc : Subsystem
      settings: PortSchema="{\"entries\":[{\"content\":{\"sides\":[{\"content\":{\"connectorIds\":[\"Out1\",\"LConn1\"]},\"type\":\"ConnectorPlacement.EquallySpacedRectSide\",\"uuid\":\"95ca4545-c473-4e31-844b-c43557042c16\"},{\"content\":{\"connectorIds\":[\"RConn1\"],\"side\":\"RIGHT\"},\"type\":\"ConnectorPlacement.EquallySpacedRectSide\",\"uuid\":\"f9304c30-8684-4a05-a34b-3121610e628d\"},{\"content\":{\"connectorIds\":[],\"side\":\"TOP\"},\"type\":\"ConnectorPlacement.EquallySpacedRectSide\",\"uuid\":\"64c7a4d8-8539-4303-ae81-4015bd1451af\"}]},\"type\":\"ConnectorPlacement.EquallySpacedConnector\",\"uuid\":\"40c12b2f-fb9d-4a19-b6f1-e93ae1fd4d68\"}],\"packageUris\":[\"http://schema.mathworks.com/mf0/Connector/R2020b\"],\"version\":\"1.0\"}"
  XenonCalc : Subsystem  mask{Volume=Volume, Area=Area, Length=Length, Dh=Dh, Elevation=Elevation}
      mask prompts: Dh "Hydraulic Diameter"
      settings: PortSchema="{\"entries\":[{\"content\":{\"sides\":[{\"content\":{\"connectorIds\":[\"LConn1\",\"In1\"]},\"type\":\"ConnectorPlacement.EquallySpacedRectSide\",\"uuid\":\"82f8e7e7-fd89-4597-952e-64db268d0190\"},{\"content\":{\"connectorIds\":[\"RConn1\",\"Out1\"],\"side\":\"RIGHT\"},\"type\":\"ConnectorPlacement.EquallySpacedRectSide\",\"uuid\":\"4b3edad1-18f8-43fa-96ee-a24bb3384b59\"},{\"content\":{\"connectorIds\":[\"In2\"],\"side\":\"TOP\"},\"type\":\"ConnectorPlacement.EquallySpacedRectSide\",\"uuid\":\"43d4f51d-f841-40d6-804e-7f238a90dabe\"},{\"content\":{\"connectorIds\":[\"In3\"],\"side\":\"BOTTOM\"},\"type\":\"ConnectorPlacement.EquallySpacedRectSide\",\"uuid\":\"350f2274-4108-4e6e-a637-0ae7118de3f0\"}]},\"type\":\"ConnectorPlacement.EquallySpacedConnector\",\"uuid\":\"d7e795ea-9d5d-4a8c-83ab-dab42197cc2f\"}],\"packageUris\":[\"http://schema.mathworks.com/mf0/Connector/R2020b\"],\"version\":\"1.0\"}"
  Inlet : PMIOPort  Side=Left
  Outlet : PMIOPort  Port=2  Side=Right
  XeOut : Outport
  GasOut : Outport  Port=2
  wires:
  XenonCalc/1(XeOut) -> XeOut/1
  Add/1 -> Gain/1
  GasCalc/1(GasOut) -> GasOut/1, Add/2
  Gain/1 -> Delay One Step/1
  GasIn/1 -> GasCalc/1(GasIn), Add/1
  Delay One Step/1 -> XenonCalc/3(GasRef), InletDistributor/1(GasInRef)
  XeIn/1 -> XenonCalc/1(XeIn)
  PLossFunc/1(PLoss) -> XenonCalc/2(PLoss)
  connections:
  Inlet/RConn1 -- GasCalc/LConn1 -- XenonCalc/LConn1
  GasCalc/LConn2 -- InletDistributor/RConn2
  Outlet/RConn1 -- PLossFunc/RConn1 -- InletDistributor/RConn1 -- GasCalc/LConn3
  InletDistributor/LConn1 -- PLossFunc/LConn1 -- XenonCalc/RConn1

== system MSREPrimaryLoop_PlantLevel/Reactor/CoreTH&Inerti/LowerPlenum ==
  XeIn : Inport
  GasIn : Inport  Port=2
  Add : Sum  Inputs=|++
  Delay One Step : Delay  DelayLength=1
  Downcomer : Subsystem
      settings: PortSchema="{\"entries\":[{\"content\":{\"sides\":[{\"content\":{\"connectorIds\":[\"LConn1\",\"In1\"]},\"type\":\"ConnectorPlacement.EquallySpacedRectSide\",\"uuid\":\"0f255306-ec83-4423-ac41-a2708bd1ec44\"},{\"content\":{\"connectorIds\":[\"RConn1\",\"RConn2\"],\"side\":\"RIGHT\"},\"type\":\"ConnectorPlacement.EquallySpacedRectSide\",\"uuid\":\"650fb4ea-7b32-4c45-8538-9785d9ca64bf\"},{\"content\":{\"side\":\"TOP\"},\"type\":\"ConnectorPlacement.EquallySpacedRectSide\",\"uuid\":\"434d3568-54a4-4787-a287-69f15ef478cb\"},{\"content\":{\"connectorIds\":[\"RConn3\",\"RConn4\"],\"side\":\"BOTTOM\"},\"type\":\"ConnectorPlacement.EquallySpacedRectSide\",\"uuid\":\"5b0b510d-1175-4508-bbe9-65b563e28484\"}]},\"type\":\"ConnectorPlacement.EquallySpacedConnector\",\"uuid\":\"b18d9c84-3d71-444b-a89d-79c3dc70d4d9\"}],\"packageUris\":[\"http://schema.mathworks.com/mf0/Connector/R2020b\"],\"version\":\"1.0\"}"
  Gain : Gain  Gain=0.5
  GasCalc : Subsystem  mask{Volume=Volume}
      settings: PortSchema="{\"entries\":[{\"content\":{\"sides\":[{\"content\":{\"connectorIds\":[\"In1\"]},\"type\":\"ConnectorPlacement.EquallySpacedRectSide\",\"uuid\":\"a8e1ce06-71c9-462d-8d5c-7a3e078b5544\"},{\"content\":{\"connectorIds\":[\"Out1\"],\"side\":\"RIGHT\"},\"type\":\"ConnectorPlacement.EquallySpacedRectSide\",\"uuid\":\"2c63a1ce-15e2-4b17-a432-f9f40781bd58\"},{\"content\":{\"connectorIds\":[\"LConn1\",\"LConn2\",\"LConn3\"],\"side\":\"TOP\"},\"type\":\"ConnectorPlacement.EquallySpacedRectSide\",\"uuid\":\"abc20e07-15eb-475f-be7f-cc96378523a1\"},{\"content\":{\"connectorIds\":[],\"side\":\"BOTTOM\"},\"type\":\"ConnectorPlacement.EquallySpacedRectSide\",\"uuid\":\"ab58f362-f4c2-4e86-bda0-802426066295\"}]},\"type\":\"ConnectorPlacement.EquallySpacedConnector\",\"uuid\":\"b54d49a9-048b-4912-bf18-92a7ef5e8aff\"}],\"packageUris\":[\"http://schema.mathworks.com/mf0/Connector/R2020b\"],\"version\":\"1.0\"}"
  PLossFunc : Subsystem
      settings: PortSchema="{\"entries\":[{\"content\":{\"sides\":[{\"content\":{\"connectorIds\":[\"Out1\",\"LConn1\"]},\"type\":\"ConnectorPlacement.EquallySpacedRectSide\",\"uuid\":\"95ca4545-c473-4e31-844b-c43557042c16\"},{\"content\":{\"connectorIds\":[\"RConn1\"],\"side\":\"RIGHT\"},\"type\":\"ConnectorPlacement.EquallySpacedRectSide\",\"uuid\":\"f9304c30-8684-4a05-a34b-3121610e628d\"},{\"content\":{\"connectorIds\":[],\"side\":\"TOP\"},\"type\":\"ConnectorPlacement.EquallySpacedRectSide\",\"uuid\":\"64c7a4d8-8539-4303-ae81-4015bd1451af\"}]},\"type\":\"ConnectorPlacement.EquallySpacedConnector\",\"uuid\":\"40c12b2f-fb9d-4a19-b6f1-e93ae1fd4d68\"}],\"packageUris\":[\"http://schema.mathworks.com/mf0/Connector/R2020b\"],\"version\":\"1.0\"}"
  XenonCalc : Subsystem  mask{Volume=Volume, Area=Area, Length=Length, Dh=Dh, Elevation=Elevation}
      mask prompts: Dh "Hydraulic Diameter"
      settings: PortSchema="{\"entries\":[{\"content\":{\"sides\":[{\"content\":{\"connectorIds\":[\"LConn1\",\"In1\"]},\"type\":\"ConnectorPlacement.EquallySpacedRectSide\",\"uuid\":\"82f8e7e7-fd89-4597-952e-64db268d0190\"},{\"content\":{\"connectorIds\":[\"RConn1\",\"Out1\"],\"side\":\"RIGHT\"},\"type\":\"ConnectorPlacement.EquallySpacedRectSide\",\"uuid\":\"4b3edad1-18f8-43fa-96ee-a24bb3384b59\"},{\"content\":{\"connectorIds\":[\"In2\"],\"side\":\"TOP\"},\"type\":\"ConnectorPlacement.EquallySpacedRectSide\",\"uuid\":\"43d4f51d-f841-40d6-804e-7f238a90dabe\"},{\"content\":{\"connectorIds\":[\"In3\"],\"side\":\"BOTTOM\"},\"type\":\"ConnectorPlacement.EquallySpacedRectSide\",\"uuid\":\"350f2274-4108-4e6e-a637-0ae7118de3f0\"}]},\"type\":\"ConnectorPlacement.EquallySpacedConnector\",\"uuid\":\"d7e795ea-9d5d-4a8c-83ab-dab42197cc2f\"}],\"packageUris\":[\"http://schema.mathworks.com/mf0/Connector/R2020b\"],\"version\":\"1.0\"}"
  Inlet : PMIOPort  Side=Left
  Outlet : PMIOPort  Port=2  Side=Right
  Thermal : PMIOPort  Port=3  Side=Left
  XeOut : Outport
  GasOut : Outport  Port=2
  wires:
  XenonCalc/1(XeOut) -> XeOut/1
  Add/1 -> Gain/1
  GasCalc/1(GasOut) -> GasOut/1, Add/2
  Gain/1 -> Delay One Step/1
  GasIn/1 -> GasCalc/1(GasIn), Add/1
  Delay One Step/1 -> XenonCalc/3(GasRef), Downcomer/1(GasInRef)
  XeIn/1 -> XenonCalc/1(XeIn)
  PLossFunc/1(PLoss) -> XenonCalc/2(PLoss)
  connections:
  Inlet/RConn1 -- GasCalc/LConn1 -- XenonCalc/LConn1
  Outlet/RConn1 -- PLossFunc/RConn1 -- GasCalc/LConn3 -- Downcomer/RConn2
  GasCalc/LConn2 -- Downcomer/RConn3
  XenonCalc/RConn1 -- PLossFunc/LConn1 -- Downcomer/LConn1
  Downcomer/RConn1 -- Thermal/RConn1

== system MSREPrimaryLoop_PlantLevel/Reactor/CoreTH&Inerti/UpperPlenum ==
  XeIn : Inport
  GasIn : Inport  Port=2
  Add : Sum  Inputs=|++
  Delay One Step : Delay  DelayLength=1
  Downcomer : Subsystem
      settings: PortSchema="{\"entries\":[{\"content\":{\"sides\":[{\"content\":{\"connectorIds\":[\"LConn1\",\"In1\"]},\"type\":\"ConnectorPlacement.EquallySpacedRectSide\",\"uuid\":\"0f255306-ec83-4423-ac41-a2708bd1ec44\"},{\"content\":{\"connectorIds\":[\"RConn1\",\"RConn2\"],\"side\":\"RIGHT\"},\"type\":\"ConnectorPlacement.EquallySpacedRectSide\",\"uuid\":\"650fb4ea-7b32-4c45-8538-9785d9ca64bf\"},{\"content\":{\"connectorIds\":[],\"side\":\"TOP\"},\"type\":\"ConnectorPlacement.EquallySpacedRectSide\",\"uuid\":\"434d3568-54a4-4787-a287-69f15ef478cb\"},{\"content\":{\"connectorIds\":[\"RConn3\"],\"side\":\"BOTTOM\"},\"type\":\"ConnectorPlacement.EquallySpacedRectSide\",\"uuid\":\"5b0b510d-1175-4508-bbe9-65b563e28484\"}]},\"type\":\"ConnectorPlacement.EquallySpacedConnector\",\"uuid\":\"b18d9c84-3d71-444b-a89d-79c3dc70d4d9\"}],\"packageUris\":[\"http://schema.mathworks.com/mf0/Connector/R2020b\"],\"version\":\"1.0\"}"
  Gain : Gain  Gain=0.5
  GasCalc : Subsystem  mask{Volume=Volume}
      settings: PortSchema="{\"entries\":[{\"content\":{\"sides\":[{\"content\":{\"connectorIds\":[\"In1\"]},\"type\":\"ConnectorPlacement.EquallySpacedRectSide\",\"uuid\":\"a8e1ce06-71c9-462d-8d5c-7a3e078b5544\"},{\"content\":{\"connectorIds\":[\"Out1\"],\"side\":\"RIGHT\"},\"type\":\"ConnectorPlacement.EquallySpacedRectSide\",\"uuid\":\"2c63a1ce-15e2-4b17-a432-f9f40781bd58\"},{\"content\":{\"connectorIds\":[\"LConn1\",\"LConn2\",\"LConn3\"],\"side\":\"TOP\"},\"type\":\"ConnectorPlacement.EquallySpacedRectSide\",\"uuid\":\"abc20e07-15eb-475f-be7f-cc96378523a1\"},{\"content\":{\"connectorIds\":[],\"side\":\"BOTTOM\"},\"type\":\"ConnectorPlacement.EquallySpacedRectSide\",\"uuid\":\"ab58f362-f4c2-4e86-bda0-802426066295\"}]},\"type\":\"ConnectorPlacement.EquallySpacedConnector\",\"uuid\":\"b54d49a9-048b-4912-bf18-92a7ef5e8aff\"}],\"packageUris\":[\"http://schema.mathworks.com/mf0/Connector/R2020b\"],\"version\":\"1.0\"}"
  PLossFunc : Subsystem
      settings: PortSchema="{\"entries\":[{\"content\":{\"sides\":[{\"content\":{\"connectorIds\":[\"Out1\",\"LConn1\"]},\"type\":\"ConnectorPlacement.EquallySpacedRectSide\",\"uuid\":\"95ca4545-c473-4e31-844b-c43557042c16\"},{\"content\":{\"connectorIds\":[\"RConn1\"],\"side\":\"RIGHT\"},\"type\":\"ConnectorPlacement.EquallySpacedRectSide\",\"uuid\":\"f9304c30-8684-4a05-a34b-3121610e628d\"},{\"content\":{\"connectorIds\":[],\"side\":\"TOP\"},\"type\":\"ConnectorPlacement.EquallySpacedRectSide\",\"uuid\":\"64c7a4d8-8539-4303-ae81-4015bd1451af\"}]},\"type\":\"ConnectorPlacement.EquallySpacedConnector\",\"uuid\":\"40c12b2f-fb9d-4a19-b6f1-e93ae1fd4d68\"}],\"packageUris\":[\"http://schema.mathworks.com/mf0/Connector/R2020b\"],\"version\":\"1.0\"}"
  XenonCalc : Subsystem  mask{Volume=Volume, Area=Area, Length=Length, Dh=Dh, Elevation=Elevation}
      mask prompts: Dh "Hydraulic Diameter"
      settings: PortSchema="{\"entries\":[{\"content\":{\"sides\":[{\"content\":{\"connectorIds\":[\"LConn1\",\"In1\"]},\"type\":\"ConnectorPlacement.EquallySpacedRectSide\",\"uuid\":\"82f8e7e7-fd89-4597-952e-64db268d0190\"},{\"content\":{\"connectorIds\":[\"RConn1\",\"Out1\"],\"side\":\"RIGHT\"},\"type\":\"ConnectorPlacement.EquallySpacedRectSide\",\"uuid\":\"4b3edad1-18f8-43fa-96ee-a24bb3384b59\"},{\"content\":{\"connectorIds\":[\"In2\"],\"side\":\"TOP\"},\"type\":\"ConnectorPlacement.EquallySpacedRectSide\",\"uuid\":\"43d4f51d-f841-40d6-804e-7f238a90dabe\"},{\"content\":{\"connectorIds\":[\"In3\"],\"side\":\"BOTTOM\"},\"type\":\"ConnectorPlacement.EquallySpacedRectSide\",\"uuid\":\"350f2274-4108-4e6e-a637-0ae7118de3f0\"}]},\"type\":\"ConnectorPlacement.EquallySpacedConnector\",\"uuid\":\"d7e795ea-9d5d-4a8c-83ab-dab42197cc2f\"}],\"packageUris\":[\"http://schema.mathworks.com/mf0/Connector/R2020b\"],\"version\":\"1.0\"}"
  Inlet : PMIOPort  Side=Left
  Outlet : PMIOPort  Port=2  Side=Right
  Thermal : PMIOPort  Port=3  Side=Left
  XeOut : Outport
  GasOut : Outport  Port=2
  wires:
  XenonCalc/1(XeOut) -> XeOut/1
  Add/1 -> Gain/1
  GasCalc/1(GasOut) -> GasOut/1, Add/2
  Gain/1 -> Delay One Step/1
  GasIn/1 -> GasCalc/1(GasIn), Add/1
  Delay One Step/1 -> XenonCalc/3(GasRef), Downcomer/1(GasInRef)
  XeIn/1 -> XenonCalc/1(XeIn)
  PLossFunc/1(PLoss) -> XenonCalc/2(PLoss)
  connections:
  Inlet/RConn1 -- XenonCalc/LConn1 -- GasCalc/LConn1
  Outlet/RConn1 -- PLossFunc/RConn1 -- GasCalc/LConn3 -- Downcomer/RConn2
  GasCalc/LConn2 -- Downcomer/RConn3
  PLossFunc/LConn1 -- XenonCalc/RConn1 -- Downcomer/LConn1
  Downcomer/RConn1 -- Thermal/RConn1

== system MSREPrimaryLoop_PlantLevel/Reactor/Decay Heat/Decay Heat ==
  note: The PHX is not included in decay heat generation, the heat is put to the rest of the reactor using a scale factor
  note: Reference from UTK MSDR model
  (n/n_0) : Inport
  Decay Power Percentage : Fcn  Expr=u(2)+u(3)+u(4)
  Decay Precursor G1 : Fcn  Expr=u(1)*Fiss_factor*gamma0 - lambda0*u(2)
  Decay Precursor G2 : Fcn  Expr=u(1)*Fiss_factor*gamma1 - lambda1*u(3)
  Decay Precursor G3 : Fcn  Expr=u(1)*Fiss_factor*gamma2 - lambda2*u(4)
  Integrator : Integrator  InitialCondition=0.025125
  Integrator1 : Integrator  InitialCondition=0.0198578
  Integrator2 : Integrator  InitialCondition=0.0227606
  Mux : Mux
      settings: DisplayOption=signals
  scale : Gain  Gain=decayScale
  "Relative Decay Power " : Outport  VectorParamsAs1DForOutWhenUnconnected=off
  tag scope: relativeDecayFraction=global
  wires:
  Decay Power Percentage/1 -> scale/1, "Relative Decay Power "/1
  Decay Precursor G1/1 -> Integrator/1
  Decay Precursor G2/1 -> Integrator1/1
  Decay Precursor G3/1 -> Integrator2/1
  Mux/1 -> Decay Precursor G3/1, Decay Precursor G2/1, Decay Precursor G1/1, Decay Power Percentage/1
  Integrator/1 -> Mux/2
  Integrator1/1 -> Mux/3
  Integrator2/1 -> Mux/4
  (n/n_0)/1 -> Mux/1
  scale/1 -> [relativeDecayFraction]

== system MSREPrimaryLoop_PlantLevel/Reactor/Decay Heat/Decay Heat Off ==
  (n/n_0) : Inport
  Constant : Constant  Value=0
  Terminator : Terminator
  "Relative Decay Power " : Outport  VectorParamsAs1DForOutWhenUnconnected=off
  tag scope: relativeDecayFraction=global
  wires:
  (n/n_0)/1 -> Terminator/1
  Constant/1 -> [relativeDecayFraction], "Relative Decay Power "/1

== system MSREPrimaryLoop_PlantLevel/Reactor/Reactivity&PKE/Ideal ==
  FlowFrac : Inport
  CORE TEMPERATURE : Inport  Port=2
  "XeCore, [cm^2]" : Inport  Port=3
  Core Void : Inport  Port=4
  Gain : Gain
  Step : Step  Time=250000  Before=1  After=0  SampleTime=0
  Terminator{,1..3} (4 alike) : Terminator
  FRACTIONAL NEUTRON DENSITY : Outport
  wires:
  CORE TEMPERATURE/1 -> Terminator/1
  "XeCore, [cm^2]"/1 -> Terminator1/1
  FlowFrac/1 -> Terminator2/1
  Gain/1 -> FRACTIONAL NEUTRON DENSITY/1
  Step/1 -> Gain/1
  Core Void/1 -> Terminator3/1

== system MSREPrimaryLoop_PlantLevel/Reactor/Reactivity&PKE/Reactivity&PKE ==
  FlowFrac : Inport
  CORE TEMPERATURE : Inport  Port=2
  "XeCore, [cm^2]" : Inport  Port=3
  Core Void : Inport  Port=4
  Acceleratred Stiff System Solver : Subsystem  VariantControl=Stiff
  REACTIVITY : Subsystem
      settings: PortSchema="{\"entries\":[{\"content\":{\"sides\":[{\"content\":{\"connectorIds\":[\"In1\",\"In2\",\"In3\"]},\"type\":\"ConnectorPlacement.EquallySpacedRectSide\",\"uuid\":\"26ed18f9-521e-467a-8165-f91acdea59eb\"},{\"content\":{\"connectorIds\":[\"Out1\"],\"side\":\"RIGHT\"},\"type\":\"ConnectorPlacement.EquallySpacedRectSide\",\"uuid\":\"cdbabf16-95d7-4a8a-8589-d756110a110a\"},{\"content\":{\"side\":\"TOP\"},\"type\":\"ConnectorPlacement.EquallySpacedRectSide\",\"uuid\":\"d0e29e64-a56b-43ad-b460-16ed8821da85\"},{\"content\":{\"connectorIds\":[\"In4\"],\"side\":\"BOTTOM\"},\"type\":\"ConnectorPlacement.EquallySpacedRectSide\",\"uuid\":\"b0e3ee0c-d165-4d95-a563-1f49b7a55c7b\"}]},\"type\":\"ConnectorPlacement.EquallySpacedConnector\",\"uuid\":\"3367cf9a-8030-444c-bb96-bbcb6f025241\"}],\"packageUris\":[\"http://schema.mathworks.com/mf0/Connector/R2020b\"],\"version\":\"1.0\"}"
  Xe and Sm : Subsystem
  FRACTIONAL NEUTRON DENSITY : Outport
  wires:
  CORE TEMPERATURE/1 -> REACTIVITY/2(CORE TEMPERATURE)
  Xe and Sm/1(Poison Level) -> REACTIVITY/3(Poison Level)
  "XeCore, [cm^2]"/1 -> Xe and Sm/1("XeCore, [cm^2]")
  REACTIVITY/1(TOTAL REACTIVITY FEEDBACK) -> Acceleratred Stiff System Solver/1(REACTIVITY)
  FlowFrac/1 -> Acceleratred Stiff System Solver/2(FLOW FRACTION)
  Acceleratred Stiff System Solver/1(FRACTIONAL NEUTRON DENSITY) -> FRACTIONAL NEUTRON DENSITY/1, REACTIVITY/4(P), Xe and Sm/2(NeutronFraction)
  Core Void/1 -> REACTIVITY/1(Core Void)
